simulink model "deney4VA"  (R2023a)
settings: Solver=VariableStepAuto  StartTime=0.0  StopTime=10  RelTol=1e-3
libraries: dspfdesign x1, commrandsrc3 x1
settings Model: Creator=ALKAN  LastModifiedBy=ALKAN

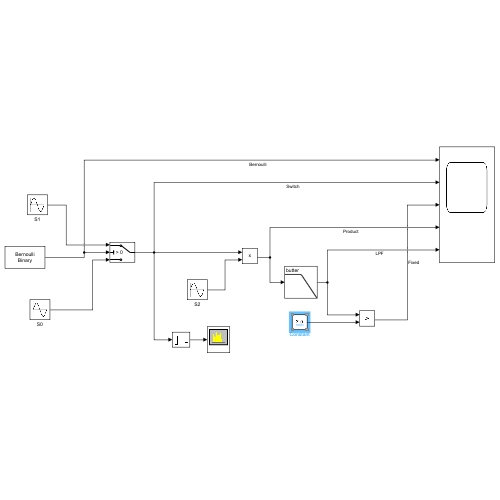
[thumbnail: Simulink's stored preview of the top-level diagram]
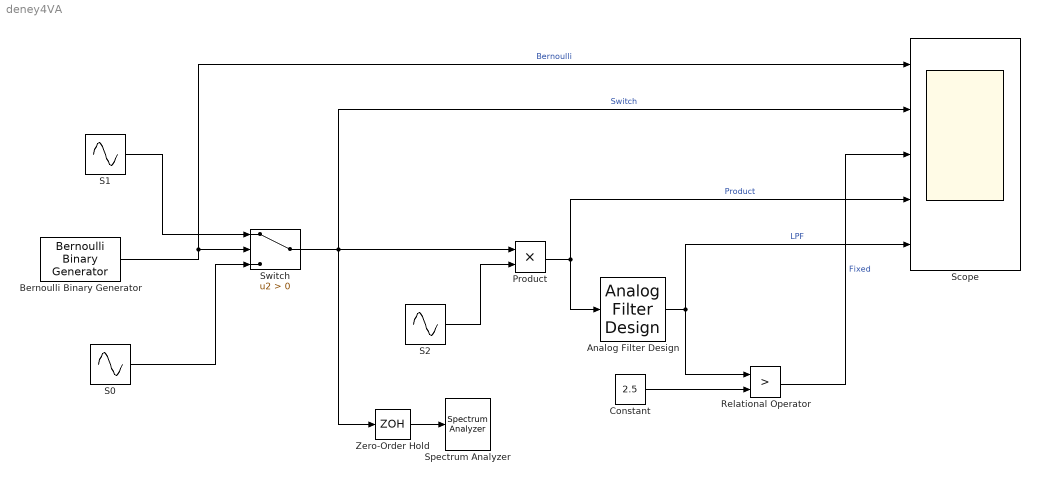
== system deney4VA ==
  Analog Filter Design : dspfdesign/Analog Filter Design  method=Butterworth  filttype=Lowpass  N=8  Wlo=1.5*2*pi  Whi=80  Rp=2  Rs=40
  Bernoulli Binary Generator : commrandsrc3/Bernoulli Binary Generator  ProbabilityOfZero=0.5  SeedSource=Auto  Seed=0  SampleTime=1  SamplesPerFrame=1  OutputDataType=double  SimulateUsing=Interpreted execution
  Constant : Constant  Value=2.5
  Product : Product
  Relational Operator : RelationalOperator  Operator=>  OutDataTypeStr=boolean  RndMeth=Simplest  InputSameDT=off
  S0 : Sin  Frequency=2*pi*2  Phase=pi/2  SampleTime=0
  S1 : Sin  Amplitude=4  Frequency=2*pi*2  Phase=pi/2  SampleTime=0
  S2 : Sin  Amplitude=2  Frequency=2*pi*2  Phase=pi/2  SampleTime=0
  Scope : Scope  NumInputPorts=5
  Spectrum Analyzer : SpectrumAnalyzer  WindowPosition=[1.000000,49.000000,1920.000000,1009.000000,]  Visible=on  ScopeFrameLocation=window  SampleRateSource=Property  SampleRate=44.1e3  PlotAsTwoSidedSpectrum=off  FrequencyScale=Log  FrequencySpan=Start and stop frequencies  StartFrequency=20  StopFrequency=20e3  YLimits=[-106.36488412,-15.49420293]  ColorLimits=[-20 80]  DefaultConfigurationName=spbscopes.SpectrumAnalyzerBlockCfg  IsFrequencyInputMode=0  FrequencyVectorPort=0  FrequencyVectorFromPort=0  FrequencyInputRBWPort=0  FrequencyInputRBWFromPort=0
  Switch : Switch  Criteria=u2 > Threshold  SaturateOnIntegerOverflow=off  InputSameDT=off
  Zero-Order Hold : ZeroOrderHold  SampleTime=0.001
  wires:
  Bernoulli Binary Generator/1 -> Scope/1, Switch/2  "Bernoulli"
  S1/1 -> Switch/1
  S0/1 -> Switch/3
  Switch/1 -> Zero-Order Hold/1, Scope/2, Product/1  "Switch"
  Zero-Order Hold/1 -> Spectrum Analyzer/1
  S2/1 -> Product/2
  Product/1 -> Analog Filter Design/1, Scope/4  "Product"
  Analog Filter Design/1 -> Relational Operator/1, Scope/5  "LPF"
  Constant/1 -> Relational Operator/2
  Relational Operator/1 -> Scope/3  "Fixed"
